simulink model "model_base_2fm"  (R2016b)
settings: Solver=FixedStepDiscrete  StartTime=0.0  StopTime=inf  FixedStep=sampleTime  RelTol=1e-3
PostLoadFcn:
  | % load model parameters
  | base_1fm_parameters;
  | 
  | % set requested state
  | set_param('model_base_2fm/Requested state','Value',num2str(0));
InitFcn:
  | % load model parameters
  | base_1fm_parameters;
  | 
  | % set requested state
  | set_param('model_base_2fm/Requested state','Value',num2str(0));
StartFcn:
  | % load model parameters
  | base_1fm_parameters;
  | 
  | % set requested state
  | set_param('model_base_2fm/Requested state','Value',num2str(0));
undefined symbols (not defined in the file or in its folder): FM1, Lb, Lf, Lu, sampleTime
undefined symbols (not defined in the file): FM2
libraries: simulink x21, LibraryFM x16, VariousBlocksLibrary x4, FMLibrary_v2 x1
(part 1 of 3)
settings Model: SimulationMode=external  Creator=niekbeckers  LastModifiedBy=Labuser
settings DataIOCC: LimitDataPoints=on  SaveFormat=Array
settings OptimizationCC: BlockReduction=off  BooleanDataType=off  LocalBlockOutputs=off  LifeSpan=inf
settings DebuggingCC: SaveWithParameterizedLinksMsg=none  UnderspecifiedInitializationDetection=Classic  MergeDetectMultiDrivingBlocksExec=none  SignalResolutionControl=TryResolveAllWithWarning  SFUnexpectedBacktrackingDiag=warning  SFNoUnconditionalDefaultTransitionDiag=warning  SFExecutionAtInitializationDiag=none
settings HardwareCC: ProdBitPerPointer=32  ProdBitPerSizeT=32  ProdBitPerPtrDiffT=32  ProdLargestAtomicFloat=None  ProdIntDivRoundTo=Undefined  ProdEndianess=Unspecified  ProdWordSize=32  ProdHWDeviceType=32-bit Generic  TargetBitPerPointer=64  TargetBitPerSizeT=64  TargetBitPerPtrDiffT=64  TargetLongLongMode=on  TargetIntDivRoundTo=Zero  TargetEndianess=LittleEndian  TargetWordSize=64  TargetHWDeviceType=MATLAB Host  ProdEqTarget=off
settings ModelReferenceCC: PropagateSignalLabelsOutOfModel=off
settings RTWCC: SystemTargetFile=TwinCAT.tlc  GenCodeOnly=on  MakeCommand=make_tct  TemplateMakefile=tct_msbuild.tmf  Description=TwinCAT Target  GenerateReport=on  TargetLang=C++
settings STFCustomTargetCC: CompOptLevelCompliant=on  GeneratePreprocessorConditionals=Disable all  MATLABClassNameForMDSCustomization=Simulink.SoftwareTarget.TargetSpecificTriggerConfigurationBase  SystemTargetFile=TwinCAT.tlc
settings ConfigComp: CovMetricSettings=dw  CovHtmlReporting=on  CovSaveCumulativeToWorkspaceVar=on  CovSaveSingleToWorkspaceVar=on  CovExternalEMLEnable=off  CovSFcnEnable=off

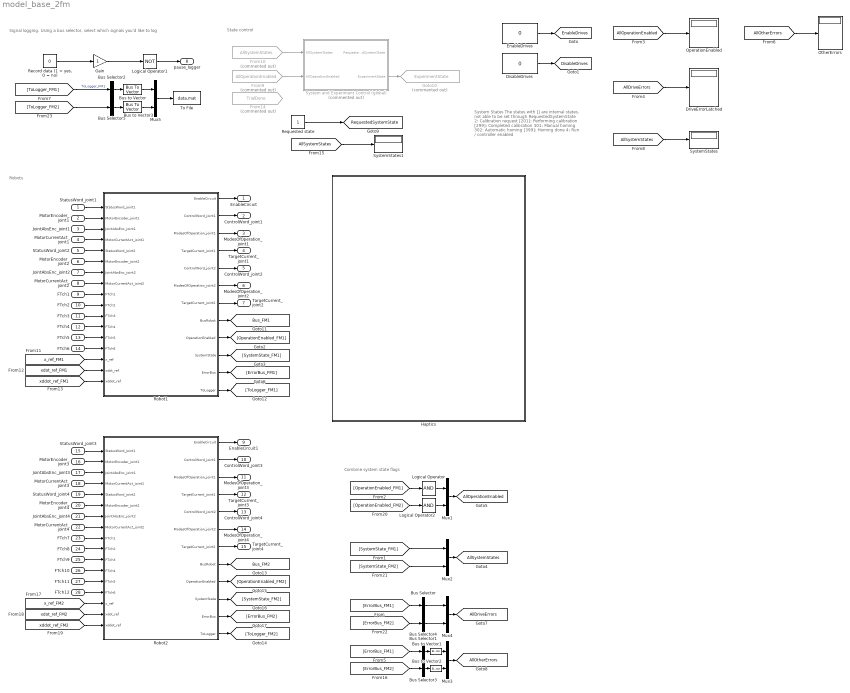
== system model_base_2fm ==
  note: Signal logging.
      | Using a bus selector, select which signals you'd like to log
  note: System States
      | The states with [] are internal states, not able to be set through RequestedSystemState
      | 2: Calibration request
      | [201]: Performing calibration
      | [299]: Completed calibration
      | 301: Manual homing
      | 302: Automatic homing
      | [399]: Homing done
      | 4: Run / controller enabled
  note: State control
  note: Combine system state flags
  note: Robots
  StatusWord_joint1 : Inport  OutDataTypeStr=uint16  PortDimensions=1
  MotorEncoder_joint1 : Inport  Port=2  OutDataTypeStr=int32  PortDimensions=1
  JointAbsEnc_joint1 : Inport  Port=3  OutDataTypeStr=int32  PortDimensions=1
  MotorCurrentAct_joint1 : Inport  Port=4  OutDataTypeStr=int16  PortDimensions=1
  StatusWord_joint2 : Inport  Port=5  OutDataTypeStr=uint16  PortDimensions=1
  MotorEncoder_joint2 : Inport  Port=6  OutDataTypeStr=int32  PortDimensions=1
  JointAbsEnc_joint2 : Inport  Port=7  OutDataTypeStr=int32  PortDimensions=1
  MotorCurrentAct_joint2 : Inport  Port=8  OutDataTypeStr=int16  PortDimensions=1
  FTch1 : Inport  Port=9  OutDataTypeStr=single  PortDimensions=1
  FTch2 : Inport  Port=10  OutDataTypeStr=single  PortDimensions=1
  FTch3 : Inport  Port=11  OutDataTypeStr=single  PortDimensions=1
  FTch4 : Inport  Port=12  OutDataTypeStr=single  PortDimensions=1
  FTch5 : Inport  Port=13  OutDataTypeStr=single  PortDimensions=1
  FTch6 : Inport  Port=14  OutDataTypeStr=single  PortDimensions=1
  StatusWord_joint3 : Inport  Port=15  OutDataTypeStr=uint16  PortDimensions=1
  MotorEncoder_joint3 : Inport  Port=16  OutDataTypeStr=int32  PortDimensions=1
  JointAbsEnc_joint3 : Inport  Port=17  OutDataTypeStr=int32  PortDimensions=1
  MotorCurrentAct_joint3 : Inport  Port=18  OutDataTypeStr=int16  PortDimensions=1
  StatusWord_joint4 : Inport  Port=19  OutDataTypeStr=uint16  PortDimensions=1
  MotorEncoder_joint4 : Inport  Port=20  OutDataTypeStr=int32  PortDimensions=1
  JointAbsEnc_joint4 : Inport  Port=21  OutDataTypeStr=int32  PortDimensions=1
  MotorCurrentAct_joint4 : Inport  Port=22  OutDataTypeStr=int16  PortDimensions=1
  FTch7 : Inport  Port=23  OutDataTypeStr=single  PortDimensions=1
  FTch8 : Inport  Port=24  OutDataTypeStr=single  PortDimensions=1
  FTch9 : Inport  Port=25  OutDataTypeStr=single  PortDimensions=1
  FTch10 : Inport  Port=26  OutDataTypeStr=single  PortDimensions=1
  FTch11 : Inport  Port=27  OutDataTypeStr=single  PortDimensions=1
  FTch12 : Inport  Port=28  OutDataTypeStr=single  PortDimensions=1
  Bus Selector : BusSelector  OutputSignals=DriveErrorLatched  OutputAsBus=on
  Bus Selector1 : BusSelector  OutputSignals=WorkspaceErrorLatched,ForceSensorLatched  OutputAsBus=on
  Bus Selector2 : BusSelector  OutputSignals=SystemState,qJointSpace.q,qJointSpace.qdot,xOpSpace.x,xOpSpace.xdot,Controller_ToLogger.x_ref,Controller_ToLogger.xdot_ref,Controller_ToLogger.xddot_ref,BusFTSensor.ForcesOpSpace,ToEtherCAT_ToLogger_Actuator1.DriveError,ToEtherCAT_ToLogger_Actuator2.DriveError,BusActuators.BusActuator1.JointVelocity_LPF_rads,BusActuators.BusActuator2.JointVelocity_LPF_rads,ToEtherCAT_ToLogger_Actuator1.DesiredTorque_Nm,ToEtherCAT_ToLogger_Actuator2.DesiredTorque_Nm,BusActuators.BusActuator1.JointPosition_AbsEnc_rad,BusActuators.BusActuator2.JointPosition_AbsEnc_rad,BusActuators.BusActuator1.JointVelocity_AbsEnc,BusActuators.BusActuator2.JointVelocity_AbsEnc  OutputAsBus=on
  Bus Selector3 : BusSelector  OutputSignals=WorkspaceErrorLatched,ForceSensorLatched  OutputAsBus=on
  Bus Selector4 : BusSelector  OutputSignals=DriveErrorLatched  OutputAsBus=on
  Bus Selector5 : BusSelector  OutputSignals=SystemState,qJointSpace.q,qJointSpace.qdot,xOpSpace.x,xOpSpace.xdot,Controller_ToLogger.x_ref,Controller_ToLogger.xdot_ref,Controller_ToLogger.xddot_ref,BusFTSensor.ForcesOpSpace,ToEtherCAT_ToLogger_Actuator1.DriveError,ToEtherCAT_ToLogger_Actuator2.DriveError,BusActuators.BusActuator1.JointVelocity_LPF_rads,BusActuators.BusActuator2.JointVelocity_LPF_rads,ToEtherCAT_ToLogger_Actuator1.DesiredTorque_Nm,ToEtherCAT_ToLogger_Actuator2.DesiredTorque_Nm,BusActuators.BusActuator1.JointPosition_AbsEnc_rad,BusActuators.BusActuator2.JointPosition_AbsEnc_rad,BusActuators.BusActuator1.JointVelocity_AbsEnc,BusActuators.BusActuator2.JointVelocity_AbsEnc  OutputAsBus=on
  Bus to Vector{,1..3} (4 alike) : BusToVector
  DisableDrives : Constant  Value=0
      settings: OpenFcn=set_param(gcb,'Value','1');tname = ['toggletimer_' gcb];delete(timerfind('name',tname));t = timer('timerfcn', ['set_param(''',gcb,''',''Value'',''0'')'],'executionmode','singleshot','startdelay',1,'name',tname);start(t);
      mask Display: fprintf('PushToTrigger\n%s',get_param(gcb,'value'))
  DriveErrorLatched : Display
  EnableDrives : Constant  Value=0
      settings: OpenFcn=set_param(gcb,'Value','1');tname = ['toggletimer_' gcb];delete(timerfind('name',tname));t = timer('timerfcn', ['set_param(''',gcb,''',''Value'',''0'')'],'executionmode','singleshot','startdelay',1,'name',tname);start(t);
      mask Display: fprintf('PushToTrigger\n%s',get_param(gcb,'value'))
  From10 : From  Commented=on  GotoTag=AllSystemStates
  From14 : From  Commented=on  GotoTag=TrialDone
  From9 : From  Commented=on  GotoTag=AllOperationEnabled
  Gain : Gain
  Goto10 : Goto  Commented=on  GotoTag=ExperimentState  TagVisibility=global
  Haptics : Subsystem
  Logical Operator : Logic  Inputs=1  AllPortsSameDT=off  OutDataTypeStr=boolean
  Logical Operator1 : Logic  Operator=NOT  Inputs=1  AllPortsSameDT=off  OutDataTypeStr=boolean
  Logical Operator2 : Logic  Inputs=1  AllPortsSameDT=off  OutDataTypeStr=boolean
  Mux{1..5} (5 alike) : Mux  Inputs=2
  OperationEnabled : Display
  OtherErrors : Display
  "Record data (1 = yes, 0 = no)" : Constant  Value=0
  Requested state : Constant
  Robot1 : Subsystem  mask{RobotStruct=FM1}
      mask prompts: RobotStruct "Robot struct (data)"
  Robot2 : Subsystem  mask{RobotStruct=FM2}
      mask prompts: RobotStruct "Robot struct (data)"
  System and Experiment Control (global) : Subsystem  Commented=on
  SystemStates : Display
  SystemStates1 : Display
  To File : ToFile  Filename=data.mat  MatrixName=data
  EnableCircuit : Outport  OutDataTypeStr=boolean  PortDimensions=1
  ControlWord_joint1 : Outport  Port=2  OutDataTypeStr=uint16  PortDimensions=1
  ModesOfOperation_joint1 : Outport  Port=3  OutDataTypeStr=int8  PortDimensions=1
  TargetCurrent_joint1 : Outport  Port=4  OutDataTypeStr=int16  PortDimensions=1
  ControlWord_joint2 : Outport  Port=5  OutDataTypeStr=uint16  PortDimensions=1
  ModesOfOperation_joint2 : Outport  Port=6  OutDataTypeStr=int8  PortDimensions=1
  TargetCurrent_joint2 : Outport  Port=7  OutDataTypeStr=int16  PortDimensions=1
  pause_logger : Outport  Port=8  OutDataTypeStr=boolean  PortDimensions=1
  EnableCircuit1 : Outport  Port=9  OutDataTypeStr=boolean  PortDimensions=1
  ControlWord_joint3 : Outport  Port=10  OutDataTypeStr=uint16  PortDimensions=1
  ModesOfOperation_joint3 : Outport  Port=11  OutDataTypeStr=int8  PortDimensions=1
  TargetCurrent_joint3 : Outport  Port=12  OutDataTypeStr=int16  PortDimensions=1
  ControlWord_joint4 : Outport  Port=13  OutDataTypeStr=uint16  PortDimensions=1
  ModesOfOperation_joint4 : Outport  Port=14  OutDataTypeStr=int8  PortDimensions=1
  TargetCurrent_joint4 : Outport  Port=15  OutDataTypeStr=int16  PortDimensions=1
  tag scope: AllDriveErrors=global, AllOperationEnabled=global, AllOtherErrors=global, AllSystemStates=global, Bus_FM1=global, Bus_FM2=global, DisableDrives=global, EnableDrives=global, RequestedSystemState=global
  wires:
  DisableDrives/1 -> [DisableDrives]
  EnableDrives/1 -> [EnableDrives]
  Robot1/9(OperationEnabled) -> [OperationEnabled_FM1]
  [AllOperationEnabled] -> OperationEnabled/1
  Robot1/10(SystemState) -> [SystemState_FM1]
  [SystemState_FM1] -> Mux2/1
  Mux2/1 -> [AllSystemStates]
  Mux1/1 -> [AllOperationEnabled]
  [OperationEnabled_FM1] -> Logical Operator/1
  Robot1/11(ErrorBus) -> [ErrorBus_FM1]
  [ErrorBus_FM1] -> Bus Selector/1
  [AllDriveErrors] -> DriveErrorLatched/1
  [ErrorBus_FM1] -> Bus Selector1/1
  [AllOtherErrors] -> OtherErrors/1
  [AllSystemStates] -> SystemStates/1
  System and Experiment Control (global)/2(ExperimentState) -> Goto10/1
  From10/1 -> System and Experiment Control (global)/1(AllSystemStates)
  From9/1 -> System and Experiment Control (global)/2(AllOperationEnabled)
  [x_ref_FM1] -> Robot1/15(x_ref)
  [xdot_ref_FM1] -> Robot1/16(xdot_ref)
  [xddot_ref_FM1] -> Robot1/17(xddot_ref)
  Requested state/1 -> [RequestedSystemState]
  Robot1/8(BusRobot) -> [Bus_FM1]
  StatusWord_joint1/1 -> Robot1/1(StatusWord_joint1)
  MotorEncoder_joint1/1 -> Robot1/2(MotorEncoder_joint1)
  JointAbsEnc_joint1/1 -> Robot1/3(JointAbsEnc_joint1)
  MotorCurrentAct_joint1/1 -> Robot1/4(MotorCurrentAct_joint1)
  StatusWord_joint2/1 -> Robot1/5(StatusWord_joint2)
  MotorEncoder_joint2/1 -> Robot1/6(MotorEncoder_joint2)
  JointAbsEnc_joint2/1 -> Robot1/7(JointAbsEnc_joint2)
  MotorCurrentAct_joint2/1 -> Robot1/8(MotorCurrentAct_joint2)
  FTch1/1 -> Robot1/9(FTch1)
  FTch2/1 -> Robot1/10(FTch2)
  FTch3/1 -> Robot1/11(FTch3)
  FTch4/1 -> Robot1/12(FTch4)
  FTch5/1 -> Robot1/13(FTch5)
  FTch6/1 -> Robot1/14(FTch6)
  Robot1/1(EnableCircuit) -> EnableCircuit/1
  Robot1/2(ControlWord_joint1) -> ControlWord_joint1/1
  Robot1/3(ModesOfOperation_joint1) -> ModesOfOperation_joint1/1
  Robot1/4(TargetCurrent_joint1) -> TargetCurrent_joint1/1
  Robot1/7(TargetCurrent_joint2) -> TargetCurrent_joint2/1
  Robot1/6(ModesOfOperation_joint2) -> ModesOfOperation_joint2/1
  Robot1/5(ControlWord_joint2) -> ControlWord_joint2/1
  Robot1/12(ToLogger) -> [ToLogger_FM1]
  [ToLogger_FM1] -> Bus Selector2/1  "ToLogger_FM1"
  Logical Operator/1 -> Mux1/1
  [AllSystemStates] -> SystemStates1/1
  Logical Operator1/1 -> pause_logger/1
  Bus Selector2/1 -> Bus to Vector/1
  "Record data (1 = yes, 0 = no)"/1 -> Gain/1
  Robot2/9(OperationEnabled) -> [OperationEnabled_FM2]
  Robot2/10(SystemState) -> [SystemState_FM2]
  Robot2/11(ErrorBus) -> [ErrorBus_FM2]
  [x_ref_FM2] -> Robot2/15(x_ref)
  [xdot_ref_FM2] -> Robot2/16(xdot_ref)
  [xddot_ref_FM2] -> Robot2/17(xddot_ref)
  Robot2/8(BusRobot) -> [Bus_FM2]
  StatusWord_joint3/1 -> Robot2/1(StatusWord_joint1)
  MotorEncoder_joint3/1 -> Robot2/2(MotorEncoder_joint1)
  JointAbsEnc_joint3/1 -> Robot2/3(JointAbsEnc_joint1)
  MotorCurrentAct_joint3/1 -> Robot2/4(MotorCurrentAct_joint1)
  StatusWord_joint4/1 -> Robot2/5(StatusWord_joint2)
  MotorEncoder_joint4/1 -> Robot2/6(MotorEncoder_joint2)
  JointAbsEnc_joint4/1 -> Robot2/7(JointAbsEnc_joint2)
  MotorCurrentAct_joint4/1 -> Robot2/8(MotorCurrentAct_joint2)
  FTch7/1 -> Robot2/9(FTch1)
  FTch8/1 -> Robot2/10(FTch2)
  FTch9/1 -> Robot2/11(FTch3)
  FTch10/1 -> Robot2/12(FTch4)
  FTch11/1 -> Robot2/13(FTch5)
  FTch12/1 -> Robot2/14(FTch6)
  Robot2/1(EnableCircuit) -> EnableCircuit1/1
  Robot2/2(ControlWord_joint1) -> ControlWord_joint3/1
  Robot2/3(ModesOfOperation_joint1) -> ModesOfOperation_joint3/1
  Robot2/4(TargetCurrent_joint1) -> TargetCurrent_joint3/1
  Robot2/7(TargetCurrent_joint2) -> TargetCurrent_joint4/1
  Robot2/6(ModesOfOperation_joint2) -> ModesOfOperation_joint4/1
  Robot2/5(ControlWord_joint2) -> ControlWord_joint4/1
  Robot2/12(ToLogger) -> [ToLogger_FM2]
  [OperationEnabled_FM2] -> Logical Operator2/1
  Logical Operator2/1 -> Mux1/2
  [SystemState_FM2] -> Mux2/2
  [ErrorBus_FM2] -> Bus Selector3/1
  Bus Selector1/1 -> Bus to Vector1/1
  Mux3/1 -> [AllOtherErrors]
  Bus to Vector1/1 -> Mux3/1
  Bus Selector3/1 -> Bus to Vector2/1
  Bus to Vector2/1 -> Mux3/2
  Mux4/1 -> [AllDriveErrors]
  Bus Selector/1 -> Mux4/1
  [ErrorBus_FM2] -> Bus Selector4/1
  Bus Selector4/1 -> Mux4/2
  [ToLogger_FM2] -> Bus Selector5/1
  Bus Selector5/1 -> Bus to Vector3/1
  Bus to Vector3/1 -> Mux5/2
  Bus to Vector/1 -> Mux5/1
  Mux5/1 -> To File/1
  Gain/1 -> Logical Operator1/1

== system model_base_2fm/Haptics ==
  note: Only run trajectory if all systems are in state 4 (run)
  Add : Sum  Commented=on
  Bus Selector : BusSelector  OutputSignals=xOpSpace.x,xOpSpace.xdot
  Bus Selector1 : BusSelector  OutputSignals=xOpSpace.x,xOpSpace.xdot
  "Check state " : simulink/Logic and Bit Operations/Compare To Constant  Commented=on  relop===  const=4  OutDataTypeStr=boolean
  Constant : Constant  Commented=on  Value=FM1.HomeLocationOpSpace
  Constant1 : Constant  Value=[0;0]
  From9 : From  Commented=on  GotoTag=ExperimentState
  Goto1 : Goto  Commented=on  GotoTag=TrialDone  TagVisibility=global
  Hypotrochoid trajectory for AFFC : Subsystem  Commented=on
  Logical Operator : Logic  Commented=on  Inputs=1  AllPortsSameDT=off  OutDataTypeStr=boolean
  Terminator1 : Terminator  Commented=on
  Terminator2 : Terminator  Commented=on
  tag scope: x_ref_FM1=global, x_ref_FM2=global, xddot_ref_FM1=global, xddot_ref_FM2=global, xdot_ref_FM1=global, xdot_ref_FM2=global
  wires:
  From9/1 -> Terminator1/1
  [Bus_FM1] -> Bus Selector/1
  Constant/1 -> Add/1
  Hypotrochoid trajectory for AFFC/1(dx_ref) -> Add/2
  Add/1 -> ?
  Hypotrochoid trajectory for AFFC/2(dxdot_ref) -> ?
  Hypotrochoid trajectory for AFFC/3(dxddot_ref) -> ?
  ? -> "Check state "/1
  "Check state "/1 -> Logical Operator/1
  Logical Operator/1 -> Hypotrochoid trajectory for AFFC/Enable
  [Bus_FM2] -> Bus Selector1/1
  Constant1/1 -> [xddot_ref_FM2], [xddot_ref_FM1]
  Bus Selector/1 -> [x_ref_FM2]  "<x>"
  Bus Selector/2 -> [xdot_ref_FM2]  "<xdot>"
  Bus Selector1/2 -> [xdot_ref_FM1]  "<xdot>"
  Bus Selector1/1 -> [x_ref_FM1]  "<x>"
  [AllSystemStates] -> Terminator2/1

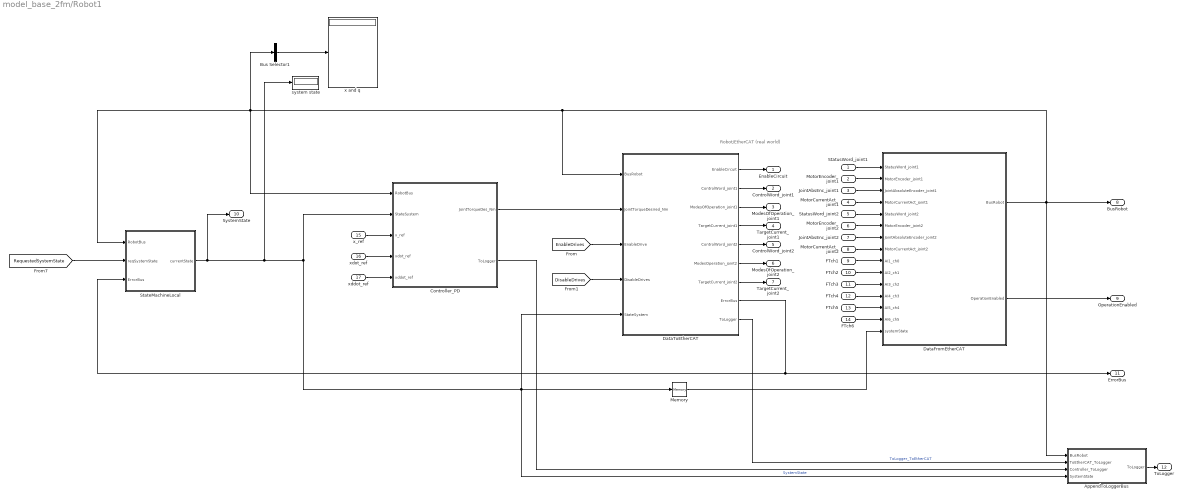
== system model_base_2fm/Robot1 ==
  note: Robot/EtherCAT (real world)
  StatusWord_joint1 : Inport
  MotorEncoder_joint1 : Inport  Port=2
  JointAbsEnc_joint1 : Inport  Port=3
  MotorCurrentAct_joint1 : Inport  Port=4
  StatusWord_joint2 : Inport  Port=5
  MotorEncoder_joint2 : Inport  Port=6
  JointAbsEnc_joint2 : Inport  Port=7
  MotorCurrentAct_joint2 : Inport  Port=8
  FTch1 : Inport  Port=9
  FTch2 : Inport  Port=10
  FTch3 : Inport  Port=11
  FTch4 : Inport  Port=12
  FTch5 : Inport  Port=13
  FTch6 : Inport  Port=14
  x_ref : Inport  Port=15
  xdot_ref : Inport  Port=16
  xddot_ref : Inport  Port=17
  AppendToLoggerBus : Subsystem
  Bus Selector1 : BusSelector  OutputSignals=qJointSpace.q,qJointSpace.qdot,xOpSpace.x,BusActuators.BusActuator1.JointPosition_AbsEnc_rad,BusActuators.BusActuator2.JointPosition_AbsEnc_rad  OutputAsBus=on
  Controller_PD : Subsystem
  DataFromEtherCAT : Subsystem
  DataToEtherCAT : Subsystem
  Memory : Memory
  StateMachineLocal : Subsystem
  system state : Display
  x and q : Display
  EnableCircuit : Outport
  ControlWord_joint1 : Outport  Port=2
  ModesOfOperation_joint1 : Outport  Port=3
  TargetCurrent_joint1 : Outport  Port=4
  ControlWord_joint2 : Outport  Port=5
  ModesOfOperation_joint2 : Outport  Port=6
  TargetCurrent_joint2 : Outport  Port=7
  BusRobot : Outport  Port=8
  OperationEnabled : Outport  Port=9
  SystemState : Outport  Port=10
  ErrorBus : Outport  Port=11
  ToLogger : Outport  Port=12
  wires:
  xddot_ref/1 -> Controller_PD/5(xddot_ref)
  xdot_ref/1 -> Controller_PD/4(xdot_ref)
  x_ref/1 -> Controller_PD/3(x_ref)
  DataToEtherCAT/7(TargetCurrent_joint2) -> TargetCurrent_joint2/1
  FTch2/1 -> DataFromEtherCAT/10(AI2_ch1)
  MotorCurrentAct_joint1/1 -> DataFromEtherCAT/4(MotorCurrentAct_joint1)
  MotorEncoder_joint2/1 -> DataFromEtherCAT/6(MotorEncoder_joint2)
  JointAbsEnc_joint1/1 -> DataFromEtherCAT/3(JointAbsoluteEncoder_joint1)
  DataToEtherCAT/3(ModesOfOperation_joint1) -> ModesOfOperation_joint1/1
  DataToEtherCAT/1(EnableCircuit) -> EnableCircuit/1
  FTch1/1 -> DataFromEtherCAT/9(AI1_ch0)
  StateMachineLocal/1(currentState) -> system state/1, DataToEtherCAT/5(StateSystem), Memory/1, AppendToLoggerBus/4(SystemState), Controller_PD/2(StateSystem), SystemState/1  "SystemState"
  DataToEtherCAT/2(ControlWord_joint1) -> ControlWord_joint1/1
  DataToEtherCAT/8(ErrorBus) -> StateMachineLocal/3(ErrorBus), ErrorBus/1
  DataFromEtherCAT/1(BusRobot) -> AppendToLoggerBus/1(BusRobot), Controller_PD/1(RobotBus), Bus Selector1/1, StateMachineLocal/1(RobotBus), DataToEtherCAT/1(BusRobot), BusRobot/1
  [RequestedSystemState] -> StateMachineLocal/2(reqSystemState)
  Controller_PD/1(JointTorqueDes_Nm) -> DataToEtherCAT/2(JointTorqueDesired_Nm)
  [DisableDrives] -> DataToEtherCAT/4(DisableDrives)
  [EnableDrives] -> DataToEtherCAT/3(EnableDrive)
  MotorCurrentAct_joint2/1 -> DataFromEtherCAT/8(MotorCurrentAct_joint2)
  DataToEtherCAT/4(TargetCurrent_joint1) -> TargetCurrent_joint1/1
  FTch5/1 -> DataFromEtherCAT/13(AI5_ch4)
  JointAbsEnc_joint2/1 -> DataFromEtherCAT/7("JointAbsoluteEncoder_joint2 ")
  MotorEncoder_joint1/1 -> DataFromEtherCAT/2(MotorEncoder_joint1)
  DataToEtherCAT/5(ControlWord_joint2) -> ControlWord_joint2/1
  DataToEtherCAT/6(ModesOperation_joint2) -> ModesOfOperation_joint2/1
  StatusWord_joint1/1 -> DataFromEtherCAT/1(StatusWord_joint1)
  StatusWord_joint2/1 -> DataFromEtherCAT/5(StatusWord_joint2)
  FTch6/1 -> DataFromEtherCAT/14(AI6_ch5)
  FTch4/1 -> DataFromEtherCAT/12(AI4_ch3)
  FTch3/1 -> DataFromEtherCAT/11(AI3_ch2)
  DataFromEtherCAT/2(OperationEnabled) -> OperationEnabled/1
  Bus Selector1/1 -> x and q/1
  Controller_PD/2(ToLogger) -> AppendToLoggerBus/3(Controller_ToLogger)
  DataToEtherCAT/9(ToLogger) -> AppendToLoggerBus/2(ToEtherCAT_ToLogger)  "ToLogger_ToEtherCAT"
  AppendToLoggerBus/1(ToLogger) -> ToLogger/1
  Memory/1 -> DataFromEtherCAT/15(systemState)

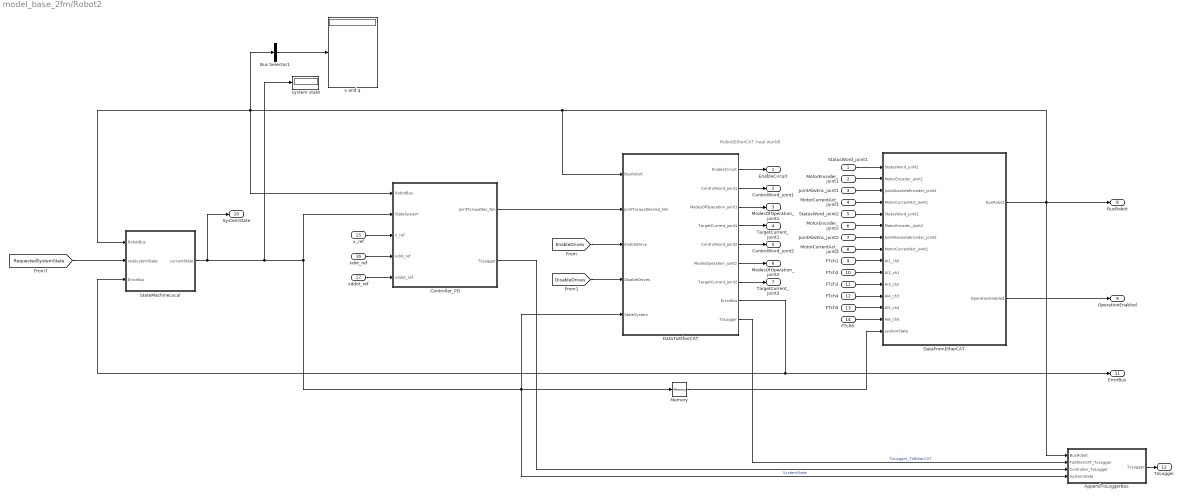
== system model_base_2fm/Robot2 ==
  note: Robot/EtherCAT (real world)
  StatusWord_joint1 : Inport
  MotorEncoder_joint1 : Inport  Port=2
  JointAbsEnc_joint1 : Inport  Port=3
  MotorCurrentAct_joint1 : Inport  Port=4
  StatusWord_joint2 : Inport  Port=5
  MotorEncoder_joint2 : Inport  Port=6
  JointAbsEnc_joint2 : Inport  Port=7
  MotorCurrentAct_joint2 : Inport  Port=8
  FTch1 : Inport  Port=9
  FTch2 : Inport  Port=10
  FTch3 : Inport  Port=11
  FTch4 : Inport  Port=12
  FTch5 : Inport  Port=13
  FTch6 : Inport  Port=14
  x_ref : Inport  Port=15
  xdot_ref : Inport  Port=16
  xddot_ref : Inport  Port=17
  AppendToLoggerBus : Subsystem
  Bus Selector1 : BusSelector  OutputSignals=qJointSpace.q,qJointSpace.qdot,xOpSpace.x,BusActuators.BusActuator1.JointPosition_AbsEnc_rad,BusActuators.BusActuator2.JointPosition_AbsEnc_rad  OutputAsBus=on
  Controller_PD : Subsystem
  DataFromEtherCAT : Subsystem
  DataToEtherCAT : Subsystem
  Memory : Memory
  StateMachineLocal : Subsystem
  system state : Display
  x and q : Display
  EnableCircuit : Outport
  ControlWord_joint1 : Outport  Port=2
  ModesOfOperation_joint1 : Outport  Port=3
  TargetCurrent_joint1 : Outport  Port=4
  ControlWord_joint2 : Outport  Port=5
  ModesOfOperation_joint2 : Outport  Port=6
  TargetCurrent_joint2 : Outport  Port=7
  BusRobot : Outport  Port=8
  OperationEnabled : Outport  Port=9
  SystemState : Outport  Port=10
  ErrorBus : Outport  Port=11
  ToLogger : Outport  Port=12
  wires:
  xddot_ref/1 -> Controller_PD/5(xddot_ref)
  xdot_ref/1 -> Controller_PD/4(xdot_ref)
  x_ref/1 -> Controller_PD/3(x_ref)
  DataToEtherCAT/7(TargetCurrent_joint2) -> TargetCurrent_joint2/1
  FTch2/1 -> DataFromEtherCAT/10(AI2_ch1)
  MotorCurrentAct_joint1/1 -> DataFromEtherCAT/4(MotorCurrentAct_joint1)
  MotorEncoder_joint2/1 -> DataFromEtherCAT/6(MotorEncoder_joint2)
  JointAbsEnc_joint1/1 -> DataFromEtherCAT/3(JointAbsoluteEncoder_joint1)
  DataToEtherCAT/3(ModesOfOperation_joint1) -> ModesOfOperation_joint1/1
  DataToEtherCAT/1(EnableCircuit) -> EnableCircuit/1
  FTch1/1 -> DataFromEtherCAT/9(AI1_ch0)
  StateMachineLocal/1(currentState) -> system state/1, DataToEtherCAT/5(StateSystem), Memory/1, AppendToLoggerBus/4(SystemState), Controller_PD/2(StateSystem), SystemState/1  "SystemState"
  DataToEtherCAT/2(ControlWord_joint1) -> ControlWord_joint1/1
  DataToEtherCAT/8(ErrorBus) -> StateMachineLocal/3(ErrorBus), ErrorBus/1
  DataFromEtherCAT/1(BusRobot) -> AppendToLoggerBus/1(BusRobot), Controller_PD/1(RobotBus), Bus Selector1/1, StateMachineLocal/1(RobotBus), DataToEtherCAT/1(BusRobot), BusRobot/1
  [RequestedSystemState] -> StateMachineLocal/2(reqSystemState)
  Controller_PD/1(JointTorqueDes_Nm) -> DataToEtherCAT/2(JointTorqueDesired_Nm)
  [DisableDrives] -> DataToEtherCAT/4(DisableDrives)
  [EnableDrives] -> DataToEtherCAT/3(EnableDrive)
  MotorCurrentAct_joint2/1 -> DataFromEtherCAT/8(MotorCurrentAct_joint2)
  DataToEtherCAT/4(TargetCurrent_joint1) -> TargetCurrent_joint1/1
  FTch5/1 -> DataFromEtherCAT/13(AI5_ch4)
  JointAbsEnc_joint2/1 -> DataFromEtherCAT/7("JointAbsoluteEncoder_joint2 ")
  MotorEncoder_joint1/1 -> DataFromEtherCAT/2(MotorEncoder_joint1)
  DataToEtherCAT/5(ControlWord_joint2) -> ControlWord_joint2/1
  DataToEtherCAT/6(ModesOperation_joint2) -> ModesOfOperation_joint2/1
  StatusWord_joint1/1 -> DataFromEtherCAT/1(StatusWord_joint1)
  StatusWord_joint2/1 -> DataFromEtherCAT/5(StatusWord_joint2)
  FTch6/1 -> DataFromEtherCAT/14(AI6_ch5)
  FTch4/1 -> DataFromEtherCAT/12(AI4_ch3)
  FTch3/1 -> DataFromEtherCAT/11(AI3_ch2)
  DataFromEtherCAT/2(OperationEnabled) -> OperationEnabled/1
  Bus Selector1/1 -> x and q/1
  Controller_PD/2(ToLogger) -> AppendToLoggerBus/3(Controller_ToLogger)
  DataToEtherCAT/9(ToLogger) -> AppendToLoggerBus/2(ToEtherCAT_ToLogger)  "ToLogger_ToEtherCAT"
  AppendToLoggerBus/1(ToLogger) -> ToLogger/1
  Memory/1 -> DataFromEtherCAT/15(systemState)

== system model_base_2fm/System and Experiment Control (global) ==
  note: Hier ergens experiment protocol inlezen
  AllSystemStates : Inport
  AllOperationEnabled : Inport  Port=2
  GlobalStateMachine : FMLibrary_v2/StateMachineLocal/SystemLocalStateMachine
  RequestedSystemState : Outport
  ExperimentState : Outport  Port=2
  wires:
  GlobalStateMachine/1 -> RequestedSystemState/1

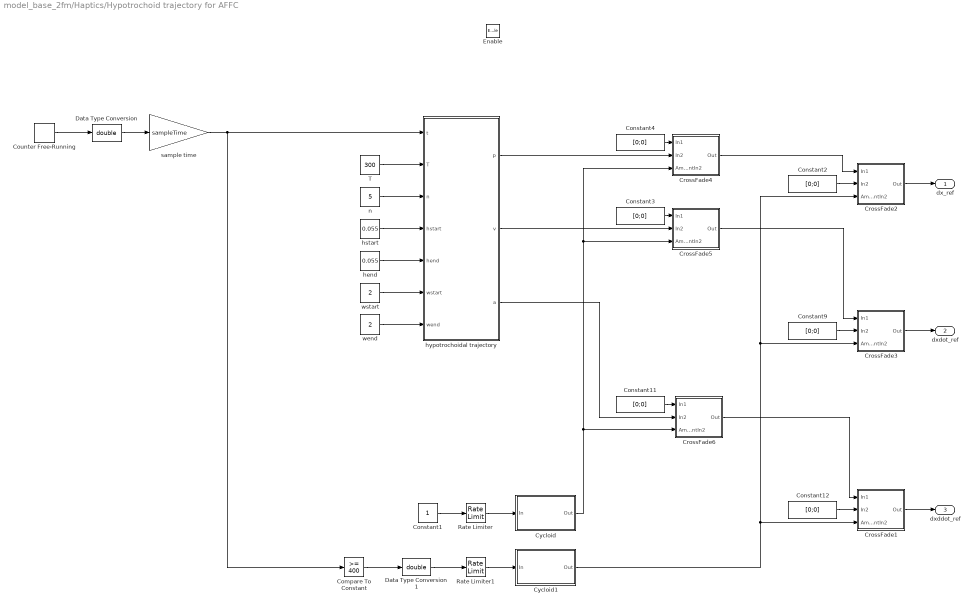
== system model_base_2fm/Haptics/Hypotrochoid trajectory for AFFC ==
  Enable : EnablePort  StatesWhenEnabling=reset
  Compare To Constant : simulink/Logic and Bit Operations/Compare To Constant  relop=>=  const=400  OutDataTypeStr=boolean
  Constant1 : Constant
  Constant{2..4,9,11..12} (6 alike) : Constant  Value=[0;0]
  Counter Free-Running : simulink/Sources/Counter Free-Running  NumBits=32  tsamp=-1
  CrossFade1 : Subsystem  AncestorBlock=VariousBlocksLibrary/Various/CrossFade
  CrossFade2 : Subsystem  AncestorBlock=VariousBlocksLibrary/Various/CrossFade
  CrossFade3 : Subsystem  AncestorBlock=VariousBlocksLibrary/Various/CrossFade
  CrossFade4 : Subsystem
  CrossFade5 : Subsystem  AncestorBlock=VariousBlocksLibrary/Various/CrossFade
  CrossFade6 : Subsystem  AncestorBlock=VariousBlocksLibrary/Various/CrossFade
  Cycloid : Subsystem  AncestorBlock=VariousBlocksLibrary/Various/Cycloid
  Cycloid1 : Subsystem  AncestorBlock=VariousBlocksLibrary/Various/Cycloid
  Data Type Conversion : DataTypeConversion  OutDataTypeStr=double
  Data Type Conversion1 : DataTypeConversion  OutDataTypeStr=double
  Rate Limiter : RateLimiter  RisingSlewLimit=0.25  FallingSlewLimit=-0.15  SampleTimeMode=inherited
  Rate Limiter1 : RateLimiter  RisingSlewLimit=0.2  FallingSlewLimit=-0.2  SampleTimeMode=inherited
  T : Constant  Value=300
  hend : Constant  Value=0.055
  hstart : Constant  Value=0.055
  hypotrochoidal trajectory : MATLAB Function  TreatAsAtomicUnit=on
  n : Constant  Value=5
  sample time : Gain  Gain=sampleTime
  wend : Constant  Value=2
  wstart : Constant  Value=2
  dx_ref : Outport  InitialOutput=[0;0]
  dxdot_ref : Outport  Port=2  InitialOutput=[0;0]
  dxddot_ref : Outport  Port=3  InitialOutput=[0;0]
  wires:
  Data Type Conversion1/1 -> Rate Limiter1/1
  hypotrochoidal trajectory/1(p) -> CrossFade4/2(In2)
  CrossFade1/1(Out) -> dxddot_ref/1
  Constant11/1 -> CrossFade6/1(In1)
  Constant12/1 -> CrossFade1/2(In2)
  CrossFade6/1(Out) -> CrossFade1/1(In1)
  Constant9/1 -> CrossFade3/2(In2)
  CrossFade5/1(Out) -> CrossFade3/1(In1)
  CrossFade3/1(Out) -> dxdot_ref/1
  Cycloid1/1(Out) -> CrossFade1/3(AmountIn2), CrossFade2/3(AmountIn2), CrossFade3/3(AmountIn2)
  Rate Limiter1/1 -> Cycloid1/1(In)
  Compare To Constant/1 -> Data Type Conversion1/1
  CrossFade4/1(Out) -> CrossFade2/1(In1)
  CrossFade2/1(Out) -> dx_ref/1
  Rate Limiter/1 -> Cycloid/1(In)
  Constant1/1 -> Rate Limiter/1
  Cycloid/1(Out) -> CrossFade6/3(AmountIn2), CrossFade5/3(AmountIn2), CrossFade4/3(AmountIn2)
  hypotrochoidal trajectory/2(v) -> CrossFade5/2(In2)
  hypotrochoidal trajectory/3(a) -> CrossFade6/2(In2)
  sample time/1 -> Compare To Constant/1, hypotrochoidal trajectory/1(t)
  Constant2/1 -> CrossFade2/2(In2)
  Data Type Conversion/1 -> sample time/1
  wstart/1 -> hypotrochoidal trajectory/6(wstart)
  wend/1 -> hypotrochoidal trajectory/7(wend)
  hstart/1 -> hypotrochoidal trajectory/4(hstart)
  hend/1 -> hypotrochoidal trajectory/5(hend)
  n/1 -> hypotrochoidal trajectory/3(n)
  T/1 -> hypotrochoidal trajectory/2(T)
  Counter Free-Running/1 -> Data Type Conversion/1
  Constant3/1 -> CrossFade5/1(In1)
  Constant4/1 -> CrossFade4/1(In1)

== system model_base_2fm/Robot1/AppendToLoggerBus ==
  BusRobot : Inport
  ToEtherCAT_ToLogger : Inport  Port=2
  Controller_ToLogger : Inport  Port=3
  SystemState : Inport  Port=4
  Bus Creator : BusCreator  Inputs=8
  Bus Selector : BusSelector  OutputSignals=xOpSpace,qJointSpace,BusFTSensor,BusActuators
  Bus Selector1 : BusSelector  OutputSignals=ToEtherCAT_ToLogger_Actuator1,ToEtherCAT_ToLogger_Actuator2
  ToLogger : Outport
  wires:
  Bus Creator/1 -> ToLogger/1  "LoggerBus"
  Bus Selector/4 -> Bus Creator/4  "<BusActuators>"
  Bus Selector/1 -> Bus Creator/1  "<xOpSpace>"
  Bus Selector/3 -> Bus Creator/3  "<BusFTSensor>"
  Bus Selector/2 -> Bus Creator/2  "<qJointSpace>"
  BusRobot/1 -> Bus Selector/1
  ToEtherCAT_ToLogger/1 -> Bus Selector1/1
  Bus Selector1/1 -> Bus Creator/5  "<ToEtherCAT_ToLogger_Actuator1>"
  Bus Selector1/2 -> Bus Creator/6  "<ToEtherCAT_ToLogger_Actuator2>"
  Controller_ToLogger/1 -> Bus Creator/7
  SystemState/1 -> Bus Creator/8  "SystemState"

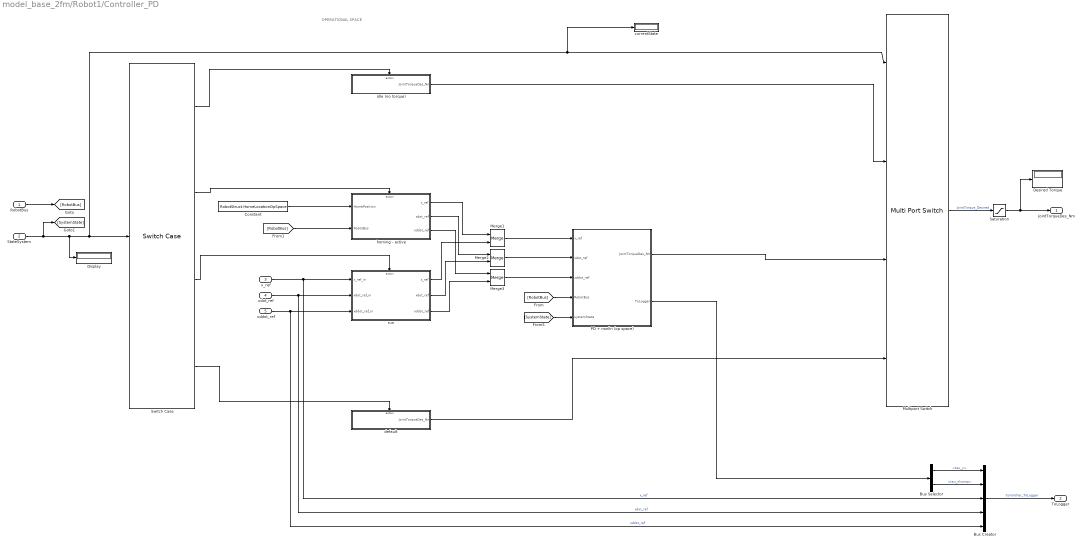
== system model_base_2fm/Robot1/Controller_PD ==
  note: OPERATIONAL SPACE
  RobotBus : Inport
  StateSystem : Inport  Port=2
  x_ref : Inport  Port=3
  xdot_ref : Inport  Port=4
  xddot_ref : Inport  Port=5
  Bus Creator : BusCreator  Inputs=5
  Bus Selector : BusSelector  OutputSignals=tau_y,tau_nlcomp
  Constant : Constant  Value=RobotStruct.HomeLocationOpSpace
  Desired Torque : Display
  Display : Display
  Merge1 : Merge  InitialOutput=[0;0]
  Merge2 : Merge  InitialOutput=[0;0]
  Merge3 : Merge  InitialOutput=[0;0]
  Multiport Switch : MultiPortSwitch  DataPortOrder=Specify indices  Inputs=4  DataPortIndices={[0,1,2,201,299,301],[302,399,4]}  DataPortForDefault=Additional data port
  PD + nonlin (op space) : Subsystem
  Saturation : Saturate  UpperLimit=4  LowerLimit=-4
  Switch Case : SwitchCase  CaseConditions={[0,1,2,201,299,301],[302, 399],[4]}
  currentState : Display
  default : Subsystem  TreatAsAtomicUnit=on
  homing - active : Subsystem
  idle (no torque) : Subsystem  TreatAsAtomicUnit=on
  run : Subsystem
  JointTorqueDes_Nm : Outport
  ToLogger : Outport  Port=2
  wires:
  [SystemState] -> PD + nonlin (op space)/5(systemState)
  xddot_ref/1 -> Bus Creator/5, run/3(xddot_ref_in)  "xddot_ref"
  xdot_ref/1 -> Bus Creator/4, run/2(xdot_ref_in)  "xdot_ref"
  x_ref/1 -> Bus Creator/3, run/1(x_ref_in)  "x_ref"
  [RobotBus] -> homing - active/2(RobotBus)
  [RobotBus] -> PD + nonlin (op space)/4(RobotBus)
  RobotBus/1 -> [RobotBus]
  PD + nonlin (op space)/1(JointTorqueDes_Nm) -> Multiport Switch/3
  Merge3/1 -> PD + nonlin (op space)/3(xddot_ref)
  Merge2/1 -> PD + nonlin (op space)/2(xdot_ref)
  Merge1/1 -> PD + nonlin (op space)/1(x_ref)
  idle (no torque)/1(JointTorqueDes_Nm) -> Multiport Switch/2
  Switch Case/2 -> homing - active/Action
  Switch Case/1 -> idle (no torque)/Action
  default/1(JointTorqueDes_Nm) -> Multiport Switch/4
  Switch Case/4 -> default/Action
  Saturation/1 -> Desired Torque/1, JointTorqueDes_Nm/1
  Switch Case/3 -> run/Action
  homing - active/1(x_ref) -> Merge1/1
  run/1(x_ref) -> Merge1/2
  StateSystem/1 -> Display/1, Multiport Switch/1, currentState/1, Switch Case/1, [SystemState]
  run/2(xdot_ref) -> Merge2/2
  run/3(xddot_ref) -> Merge3/2
  homing - active/2(xdot_ref) -> Merge2/1
  homing - active/3(xddot_ref) -> Merge3/1
  Multiport Switch/1 -> Saturation/1  "JointTorque_Desired"
  PD + nonlin (op space)/2(ToLogger) -> Bus Selector/1
  Constant/1 -> homing - active/1(HomePosition)
  Bus Creator/1 -> ToLogger/1  "Controller_ToLogger"
  Bus Selector/1 -> Bus Creator/1  "<tau_y>"
  Bus Selector/2 -> Bus Creator/2  "<tau_nlcomp>"

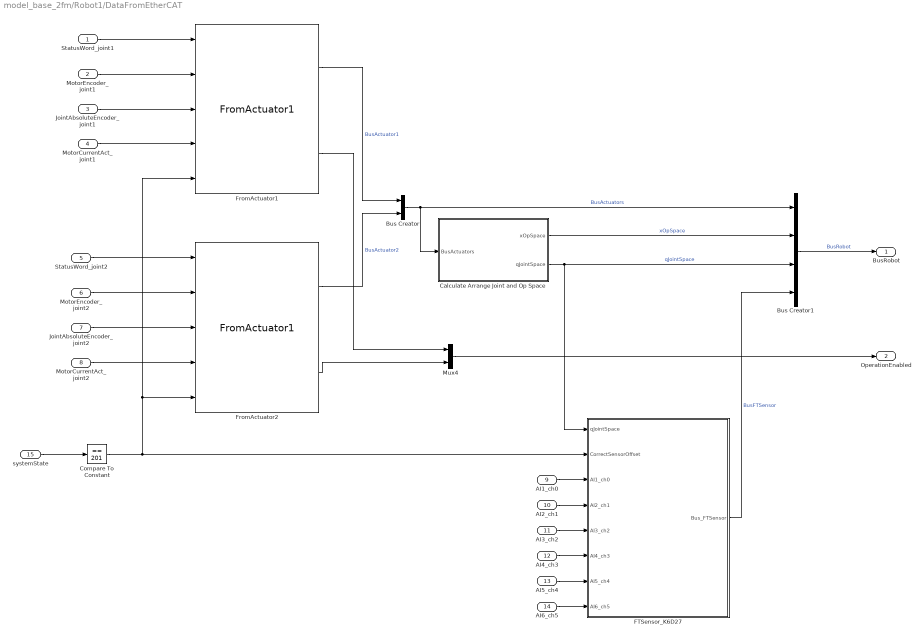
== system model_base_2fm/Robot1/DataFromEtherCAT ==
  StatusWord_joint1 : Inport
  MotorEncoder_joint1 : Inport  Port=2
  JointAbsoluteEncoder_joint1 : Inport  Port=3
  MotorCurrentAct_joint1 : Inport  Port=4
  StatusWord_joint2 : Inport  Port=5
  MotorEncoder_joint2 : Inport  Port=6
  "JointAbsoluteEncoder_joint2 " : Inport  Port=7
  MotorCurrentAct_joint2 : Inport  Port=8
  AI1_ch0 : Inport  Port=9
  AI2_ch1 : Inport  Port=10
  AI3_ch2 : Inport  Port=11
  AI4_ch3 : Inport  Port=12
  AI5_ch4 : Inport  Port=13
  AI6_ch5 : Inport  Port=14
  systemState : Inport  Port=15
  Bus Creator : BusCreator  Inputs=2
  Bus Creator1 : BusCreator  Inputs=4
  Calculate Arrange Joint and Op Space : Subsystem
  Compare To Constant : simulink/Logic and Bit Operations/Compare To Constant  relop===  const=201  OutDataTypeStr=boolean
  FTSensor_K6D27 : Subsystem  mask{FTSensorStruct=RobotStruct.FTSensor}
      mask prompts: FTSensorStruct "Struct for force torque sensor"
  FromActuator1 : LibraryFM/FromActuator1  ActuatorStruct=RobotStruct.Actuator1
  FromActuator2 : LibraryFM/FromActuator1  ActuatorStruct=RobotStruct.Actuator2
  Mux4 : Mux  Inputs=2
  BusRobot : Outport
  OperationEnabled : Outport  Port=2
  wires:
  FTSensor_K6D27/1(Bus_FTSensor) -> Bus Creator1/4  "BusFTSensor"
  FromActuator1/1 -> Bus Creator/1  "BusActuator1"
  FromActuator2/1 -> Bus Creator/2  "BusActuator2"
  FromActuator1/2 -> Mux4/1
  Mux4/1 -> OperationEnabled/1
  FromActuator2/2 -> Mux4/2
  MotorEncoder_joint1/1 -> FromActuator1/2
  StatusWord_joint1/1 -> FromActuator1/1
  JointAbsoluteEncoder_joint1/1 -> FromActuator1/3
  MotorCurrentAct_joint1/1 -> FromActuator1/4
  MotorEncoder_joint2/1 -> FromActuator2/2
  StatusWord_joint2/1 -> FromActuator2/1
  "JointAbsoluteEncoder_joint2 "/1 -> FromActuator2/3
  MotorCurrentAct_joint2/1 -> FromActuator2/4
  Bus Creator/1 -> Calculate Arrange Joint and Op Space/1(BusActuators), Bus Creator1/1  "BusActuators"
  Bus Creator1/1 -> BusRobot/1  "BusRobot"
  Calculate Arrange Joint and Op Space/2(qJointSpace) -> Bus Creator1/3, FTSensor_K6D27/1(qJointSpace)  "qJointSpace"
  systemState/1 -> Compare To Constant/1
  AI1_ch0/1 -> FTSensor_K6D27/3(AI1_ch0)
  AI2_ch1/1 -> FTSensor_K6D27/4(AI2_ch1)
  AI3_ch2/1 -> FTSensor_K6D27/5(AI3_ch2)
  AI4_ch3/1 -> FTSensor_K6D27/6(AI4_ch3)
  AI5_ch4/1 -> FTSensor_K6D27/7(AI5_ch4)
  AI6_ch5/1 -> FTSensor_K6D27/8(AI6_ch5)
  Compare To Constant/1 -> FromActuator1/5, FromActuator2/5, FTSensor_K6D27/2(CorrectSensorOffset)
  Calculate Arrange Joint and Op Space/1(xOpSpace) -> Bus Creator1/2  "xOpSpace"

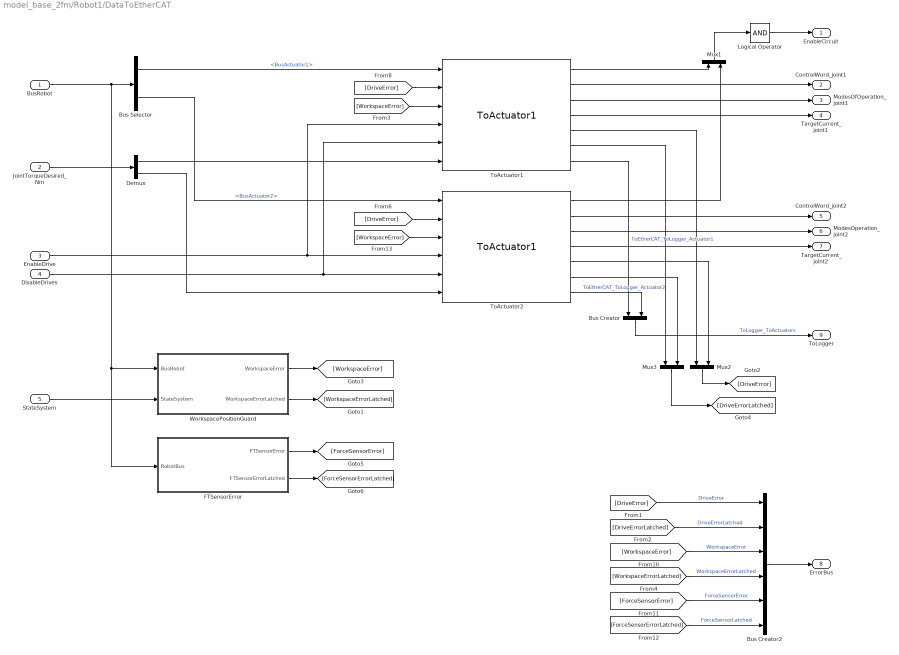
== system model_base_2fm/Robot1/DataToEtherCAT ==
  BusRobot : Inport
  JointTorqueDesired_Nm : Inport  Port=2
  EnableDrive : Inport  Port=3
  DisableDrives : Inport  Port=4
  StateSystem : Inport  Port=5
  Bus Creator : BusCreator  Inputs=2
  Bus Creator2 : BusCreator  Inputs=6
  Bus Selector : BusSelector  OutputSignals=BusActuators.BusActuator1,BusActuators.BusActuator2
  Demux : Demux  Outputs=2
  FTSensorError : Subsystem
  Logical Operator : Logic  Inputs=1  AllPortsSameDT=off  OutDataTypeStr=boolean
  Mux1 : Mux  Inputs=2
  Mux2 : Mux  Inputs=2
  Mux3 : Mux  Inputs=2
  ToActuator1 : LibraryFM/ToActuator1  ActuatorStruct=RobotStruct.Actuator1
  ToActuator2 : LibraryFM/ToActuator1  ActuatorStruct=RobotStruct.Actuator2
  WorkspacePositionGuard : Subsystem
  EnableCircuit : Outport  OutDataTypeStr=boolean
  ControlWord_joint1 : Outport  Port=2  OutDataTypeStr=uint16
  ModesOfOperation_joint1 : Outport  Port=3  OutDataTypeStr=int8
  TargetCurrent_joint1 : Outport  Port=4  OutDataTypeStr=int16
  ControlWord_joint2 : Outport  Port=5  OutDataTypeStr=uint16
  ModesOperation_joint2 : Outport  Port=6  OutDataTypeStr=int8
  TargetCurrent_joint2 : Outport  Port=7  OutDataTypeStr=int16
  ErrorBus : Outport  Port=8
  ToLogger : Outport  Port=9
  wires:
  Bus Creator/1 -> ToLogger/1  "ToLogger_ToActuators"
  ToActuator2/7 -> Bus Creator/2  "ToEtherCAT_ToLogger_Actuator2"
  ToActuator1/7 -> Bus Creator/1  "ToEtherCAT_ToLogger_Actuator1"
  ToActuator1/5 -> Mux2/1
  ToActuator2/5 -> Mux2/2
  Mux2/1 -> [DriveError]
  ToActuator1/6 -> Mux3/1
  ToActuator2/6 -> Mux3/2
  [DriveError] -> ToActuator1/2
  Mux1/1 -> Logical Operator/1
  ToActuator1/1 -> Mux1/1
  ToActuator2/1 -> Mux1/2
  ToActuator1/2 -> ControlWord_joint1/1
  ToActuator1/3 -> ModesOfOperation_joint1/1
  ToActuator2/2 -> ControlWord_joint2/1
  ToActuator1/4 -> TargetCurrent_joint1/1
  ToActuator2/4 -> TargetCurrent_joint2/1
  ToActuator2/3 -> ModesOperation_joint2/1
  Logical Operator/1 -> EnableCircuit/1
  Demux/2 -> ToActuator2/6
  JointTorqueDesired_Nm/1 -> Demux/1
  Demux/1 -> ToActuator1/6
  BusRobot/1 -> WorkspacePositionGuard/1(BusRobot), FTSensorError/1(RobotBus), Bus Selector/1
  Bus Selector/2 -> ToActuator2/1  "<BusActuator2>"
  Bus Selector/1 -> ToActuator1/1  "<BusActuator1>"
  [WorkspaceError] -> ToActuator1/3
  DisableDrives/1 -> ToActuator1/5, ToActuator2/5
  EnableDrive/1 -> ToActuator1/4, ToActuator2/4
  [DriveError] -> ToActuator2/2
  [WorkspaceError] -> ToActuator2/3
  Mux3/1 -> [DriveErrorLatched]
  Bus Creator2/1 -> ErrorBus/1
  [DriveError] -> Bus Creator2/1  "DriveError"
  [DriveErrorLatched] -> Bus Creator2/2  "DriveErrorLatched"
  [WorkspaceError] -> Bus Creator2/3  "WorkspaceError"
  [WorkspaceErrorLatched] -> Bus Creator2/4  "WorkspaceErrorLatched"
  StateSystem/1 -> WorkspacePositionGuard/2(StateSystem)
  [ForceSensorError] -> Bus Creator2/5  "ForceSensorError"
  [ForceSensorErrorLatched] -> Bus Creator2/6  "ForceSensorLatched"
  FTSensorError/1(FTSensorError) -> [ForceSensorError]
  FTSensorError/2(FTSensorErrorLatched) -> [ForceSensorErrorLatched]
  WorkspacePositionGuard/1(WorkspaceError) -> [WorkspaceError]
  WorkspacePositionGuard/2(WorkspaceErrorLatched) -> [WorkspaceErrorLatched]

== system model_base_2fm/Robot1/StateMachineLocal ==
  note: Very crude error handling
      | Ideally, the state machine gets all
      | the error codes (2,4,8, etc) such that
      | it can discern between states
  RobotBus : Inport
  reqSystemState : Inport  Port=2
  ErrorBus : Inport  Port=3
  Bus Selector : BusSelector  OutputSignals=qJointSpace.qdot,xOpSpace.x
  Bus Selector1 : BusSelector  OutputSignals=DriveError,WorkspaceError,ForceSensorError  OutputAsBus=on
  CheckVelThreshold : MATLAB Function  TreatAsAtomicUnit=on
  Compare To Constant : simulink/Logic and Bit Operations/Compare To Constant  relop=>  const=0  OutDataTypeStr=boolean
  Constant : Constant  Value=RobotStruct.HomeLocationSize
  Constant1 : Constant  Value=RobotStruct.HomeLocationOpSpace
  Constant2 : Constant  Value=0.05
  Detect Change1 : simulink/Logic and Bit Operations/Detect Change  Commented=on  vinit=0  InputProcessing=Inherited  OutDataTypeStr=boolean
  Encode system state change : MATLAB Function  Commented=on  TreatAsAtomicUnit=on
  Logical Operator : Logic  Operator=OR  Inputs=1  AllPortsSameDT=off  OutDataTypeStr=boolean
  State machine : Stateflow chart  TreatAsAtomicUnit=on
  Terminator : Terminator  Commented=on
  checkEndpointPosition : MATLAB Function  TreatAsAtomicUnit=on
  system state : Display
  currentState : Outport
  wires:
  Bus Selector1/1 -> Compare To Constant/1
  ErrorBus/1 -> Bus Selector1/1
  State machine/1(currentState) -> currentState/1, system state/1
  Logical Operator/1 -> State machine/2(fault)
  Compare To Constant/1 -> Logical Operator/1
  reqSystemState/1 -> State machine/1(requestedState)
  Detect Change1/1 -> Encode system state change/1(stateChanged)
  Encode system state change/1(systemStateChanged) -> Terminator/1
  RobotBus/1 -> Bus Selector/1
  Bus Selector/1 -> CheckVelThreshold/1(qdot)  "<qdot>"
  Bus Selector/2 -> checkEndpointPosition/1(x)  "<x>"
  CheckVelThreshold/1(velBelowThreshold) -> State machine/3(velBelowThreshold)
  Constant2/1 -> CheckVelThreshold/2(threshold)
  Constant1/1 -> checkEndpointPosition/2(homeLocation)
  Constant/1 -> checkEndpointPosition/3(threshold)
  checkEndpointPosition/1(isAtEndpoint) -> State machine/4(isAtHome)

== system model_base_2fm/Robot2/AppendToLoggerBus ==
  BusRobot : Inport
  ToEtherCAT_ToLogger : Inport  Port=2
  Controller_ToLogger : Inport  Port=3
  SystemState : Inport  Port=4
  Bus Creator : BusCreator  Inputs=8
  Bus Selector : BusSelector  OutputSignals=xOpSpace,qJointSpace,BusFTSensor,BusActuators
  Bus Selector1 : BusSelector  OutputSignals=ToEtherCAT_ToLogger_Actuator1,ToEtherCAT_ToLogger_Actuator2
  ToLogger : Outport
  wires:
  Bus Creator/1 -> ToLogger/1  "LoggerBus"
  Bus Selector/4 -> Bus Creator/4  "<BusActuators>"
  Bus Selector/1 -> Bus Creator/1  "<xOpSpace>"
  Bus Selector/3 -> Bus Creator/3  "<BusFTSensor>"
  Bus Selector/2 -> Bus Creator/2  "<qJointSpace>"
  BusRobot/1 -> Bus Selector/1
  ToEtherCAT_ToLogger/1 -> Bus Selector1/1
  Bus Selector1/1 -> Bus Creator/5  "<ToEtherCAT_ToLogger_Actuator1>"
  Bus Selector1/2 -> Bus Creator/6  "<ToEtherCAT_ToLogger_Actuator2>"
  Controller_ToLogger/1 -> Bus Creator/7
  SystemState/1 -> Bus Creator/8  "SystemState"

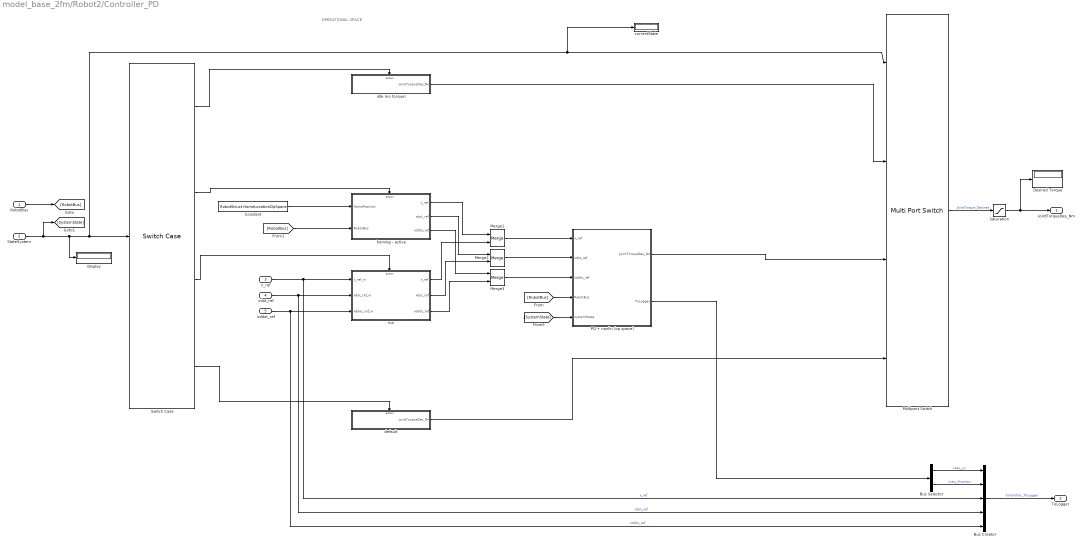
== system model_base_2fm/Robot2/Controller_PD ==
  note: OPERATIONAL SPACE
  RobotBus : Inport
  StateSystem : Inport  Port=2
  x_ref : Inport  Port=3
  xdot_ref : Inport  Port=4
  xddot_ref : Inport  Port=5
  Bus Creator : BusCreator  Inputs=5
  Bus Selector : BusSelector  OutputSignals=tau_y,tau_nlcomp
  Constant : Constant  Value=RobotStruct.HomeLocationOpSpace
  Desired Torque : Display
  Display : Display
  Merge1 : Merge  InitialOutput=[0;0]
  Merge2 : Merge  InitialOutput=[0;0]
  Merge3 : Merge  InitialOutput=[0;0]
  Multiport Switch : MultiPortSwitch  DataPortOrder=Specify indices  Inputs=4  DataPortIndices={[0,1,2,201,299,301],[302,399,4]}  DataPortForDefault=Additional data port
  PD + nonlin (op space) : Subsystem
  Saturation : Saturate  UpperLimit=4  LowerLimit=-4
  Switch Case : SwitchCase  CaseConditions={[0,1,2,201,299,301],[302, 399],[4]}
  currentState : Display
  default : Subsystem  TreatAsAtomicUnit=on
  homing - active : Subsystem
  idle (no torque) : Subsystem  TreatAsAtomicUnit=on
  run : Subsystem
  JointTorqueDes_Nm : Outport
  ToLogger : Outport  Port=2
  wires:
  [SystemState] -> PD + nonlin (op space)/5(systemState)
  xddot_ref/1 -> Bus Creator/5, run/3(xddot_ref_in)  "xddot_ref"
  xdot_ref/1 -> Bus Creator/4, run/2(xdot_ref_in)  "xdot_ref"
  x_ref/1 -> Bus Creator/3, run/1(x_ref_in)  "x_ref"
  [RobotBus] -> homing - active/2(RobotBus)
  [RobotBus] -> PD + nonlin (op space)/4(RobotBus)
  RobotBus/1 -> [RobotBus]
  PD + nonlin (op space)/1(JointTorqueDes_Nm) -> Multiport Switch/3
  Merge3/1 -> PD + nonlin (op space)/3(xddot_ref)
  Merge2/1 -> PD + nonlin (op space)/2(xdot_ref)
  Merge1/1 -> PD + nonlin (op space)/1(x_ref)
  idle (no torque)/1(JointTorqueDes_Nm) -> Multiport Switch/2
  Switch Case/2 -> homing - active/Action
  Switch Case/1 -> idle (no torque)/Action
  default/1(JointTorqueDes_Nm) -> Multiport Switch/4
  Switch Case/4 -> default/Action
  Saturation/1 -> Desired Torque/1, JointTorqueDes_Nm/1
  Switch Case/3 -> run/Action
  homing - active/1(x_ref) -> Merge1/1
  run/1(x_ref) -> Merge1/2
  StateSystem/1 -> Display/1, Multiport Switch/1, currentState/1, Switch Case/1, [SystemState]
  run/2(xdot_ref) -> Merge2/2
  run/3(xddot_ref) -> Merge3/2
  homing - active/2(xdot_ref) -> Merge2/1
  homing - active/3(xddot_ref) -> Merge3/1
  Multiport Switch/1 -> Saturation/1  "JointTorque_Desired"
  PD + nonlin (op space)/2(ToLogger) -> Bus Selector/1
  Constant/1 -> homing - active/1(HomePosition)
  Bus Creator/1 -> ToLogger/1  "Controller_ToLogger"
  Bus Selector/1 -> Bus Creator/1  "<tau_y>"
  Bus Selector/2 -> Bus Creator/2  "<tau_nlcomp>"

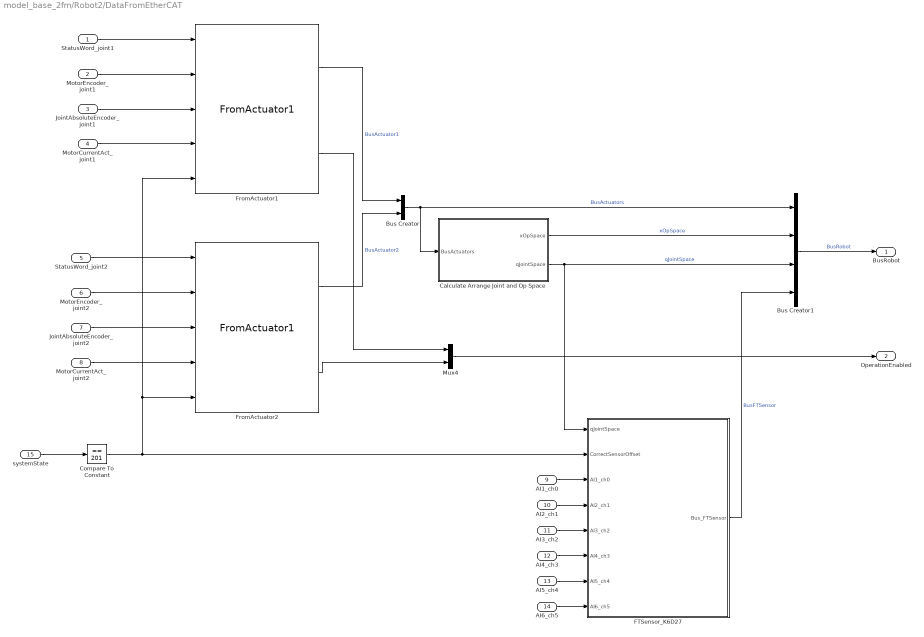
== system model_base_2fm/Robot2/DataFromEtherCAT ==
  StatusWord_joint1 : Inport
  MotorEncoder_joint1 : Inport  Port=2
  JointAbsoluteEncoder_joint1 : Inport  Port=3
  MotorCurrentAct_joint1 : Inport  Port=4
  StatusWord_joint2 : Inport  Port=5
  MotorEncoder_joint2 : Inport  Port=6
  "JointAbsoluteEncoder_joint2 " : Inport  Port=7
  MotorCurrentAct_joint2 : Inport  Port=8
  AI1_ch0 : Inport  Port=9
  AI2_ch1 : Inport  Port=10
  AI3_ch2 : Inport  Port=11
  AI4_ch3 : Inport  Port=12
  AI5_ch4 : Inport  Port=13
  AI6_ch5 : Inport  Port=14
  systemState : Inport  Port=15
  Bus Creator : BusCreator  Inputs=2
  Bus Creator1 : BusCreator  Inputs=4
  Calculate Arrange Joint and Op Space : Subsystem
  Compare To Constant : simulink/Logic and Bit Operations/Compare To Constant  relop===  const=201  OutDataTypeStr=boolean
  FTSensor_K6D27 : Subsystem  mask{FTSensorStruct=RobotStruct.FTSensor}
      mask prompts: FTSensorStruct "Struct for force torque sensor"
  FromActuator1 : LibraryFM/FromActuator1  ActuatorStruct=RobotStruct.Actuator1
  FromActuator2 : LibraryFM/FromActuator1  ActuatorStruct=RobotStruct.Actuator2
  Mux4 : Mux  Inputs=2
  BusRobot : Outport
  OperationEnabled : Outport  Port=2
  wires:
  FTSensor_K6D27/1(Bus_FTSensor) -> Bus Creator1/4  "BusFTSensor"
  FromActuator1/1 -> Bus Creator/1  "BusActuator1"
  FromActuator2/1 -> Bus Creator/2  "BusActuator2"
  FromActuator1/2 -> Mux4/1
  Mux4/1 -> OperationEnabled/1
  FromActuator2/2 -> Mux4/2
  MotorEncoder_joint1/1 -> FromActuator1/2
  StatusWord_joint1/1 -> FromActuator1/1
  JointAbsoluteEncoder_joint1/1 -> FromActuator1/3
  MotorCurrentAct_joint1/1 -> FromActuator1/4
  MotorEncoder_joint2/1 -> FromActuator2/2
  StatusWord_joint2/1 -> FromActuator2/1
  "JointAbsoluteEncoder_joint2 "/1 -> FromActuator2/3
  MotorCurrentAct_joint2/1 -> FromActuator2/4
  Bus Creator/1 -> Calculate Arrange Joint and Op Space/1(BusActuators), Bus Creator1/1  "BusActuators"
  Bus Creator1/1 -> BusRobot/1  "BusRobot"
  Calculate Arrange Joint and Op Space/2(qJointSpace) -> Bus Creator1/3, FTSensor_K6D27/1(qJointSpace)  "qJointSpace"
  systemState/1 -> Compare To Constant/1
  AI1_ch0/1 -> FTSensor_K6D27/3(AI1_ch0)
  AI2_ch1/1 -> FTSensor_K6D27/4(AI2_ch1)
  AI3_ch2/1 -> FTSensor_K6D27/5(AI3_ch2)
  AI4_ch3/1 -> FTSensor_K6D27/6(AI4_ch3)
  AI5_ch4/1 -> FTSensor_K6D27/7(AI5_ch4)
  AI6_ch5/1 -> FTSensor_K6D27/8(AI6_ch5)
  Compare To Constant/1 -> FromActuator1/5, FromActuator2/5, FTSensor_K6D27/2(CorrectSensorOffset)
  Calculate Arrange Joint and Op Space/1(xOpSpace) -> Bus Creator1/2  "xOpSpace"

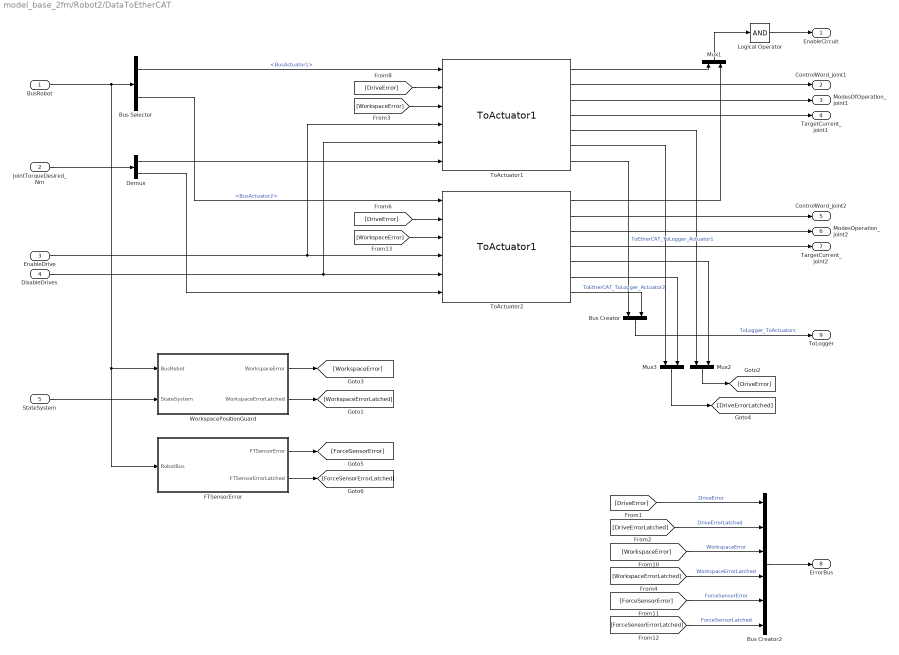
== system model_base_2fm/Robot2/DataToEtherCAT ==
  BusRobot : Inport
  JointTorqueDesired_Nm : Inport  Port=2
  EnableDrive : Inport  Port=3
  DisableDrives : Inport  Port=4
  StateSystem : Inport  Port=5
  Bus Creator : BusCreator  Inputs=2
  Bus Creator2 : BusCreator  Inputs=6
  Bus Selector : BusSelector  OutputSignals=BusActuators.BusActuator1,BusActuators.BusActuator2
  Demux : Demux  Outputs=2
  FTSensorError : Subsystem
  Logical Operator : Logic  Inputs=1  AllPortsSameDT=off  OutDataTypeStr=boolean
  Mux1 : Mux  Inputs=2
  Mux2 : Mux  Inputs=2
  Mux3 : Mux  Inputs=2
  ToActuator1 : LibraryFM/ToActuator1  ActuatorStruct=RobotStruct.Actuator1
  ToActuator2 : LibraryFM/ToActuator1  ActuatorStruct=RobotStruct.Actuator2
  WorkspacePositionGuard : Subsystem
  EnableCircuit : Outport  OutDataTypeStr=boolean
  ControlWord_joint1 : Outport  Port=2  OutDataTypeStr=uint16
  ModesOfOperation_joint1 : Outport  Port=3  OutDataTypeStr=int8
  TargetCurrent_joint1 : Outport  Port=4  OutDataTypeStr=int16
  ControlWord_joint2 : Outport  Port=5  OutDataTypeStr=uint16
  ModesOperation_joint2 : Outport  Port=6  OutDataTypeStr=int8
  TargetCurrent_joint2 : Outport  Port=7  OutDataTypeStr=int16
  ErrorBus : Outport  Port=8
  ToLogger : Outport  Port=9
  wires:
  Bus Creator/1 -> ToLogger/1  "ToLogger_ToActuators"
  ToActuator2/7 -> Bus Creator/2  "ToEtherCAT_ToLogger_Actuator2"
  ToActuator1/7 -> Bus Creator/1  "ToEtherCAT_ToLogger_Actuator1"
  ToActuator1/5 -> Mux2/1
  ToActuator2/5 -> Mux2/2
  Mux2/1 -> [DriveError]
  ToActuator1/6 -> Mux3/1
  ToActuator2/6 -> Mux3/2
  [DriveError] -> ToActuator1/2
  Mux1/1 -> Logical Operator/1
  ToActuator1/1 -> Mux1/1
  ToActuator2/1 -> Mux1/2
  ToActuator1/2 -> ControlWord_joint1/1
  ToActuator1/3 -> ModesOfOperation_joint1/1
  ToActuator2/2 -> ControlWord_joint2/1
  ToActuator1/4 -> TargetCurrent_joint1/1
  ToActuator2/4 -> TargetCurrent_joint2/1
  ToActuator2/3 -> ModesOperation_joint2/1
  Logical Operator/1 -> EnableCircuit/1
  Demux/2 -> ToActuator2/6
  JointTorqueDesired_Nm/1 -> Demux/1
  Demux/1 -> ToActuator1/6
  BusRobot/1 -> WorkspacePositionGuard/1(BusRobot), FTSensorError/1(RobotBus), Bus Selector/1
  Bus Selector/2 -> ToActuator2/1  "<BusActuator2>"
  Bus Selector/1 -> ToActuator1/1  "<BusActuator1>"
  [WorkspaceError] -> ToActuator1/3
  DisableDrives/1 -> ToActuator1/5, ToActuator2/5
  EnableDrive/1 -> ToActuator1/4, ToActuator2/4
  [DriveError] -> ToActuator2/2
  [WorkspaceError] -> ToActuator2/3
  Mux3/1 -> [DriveErrorLatched]
  Bus Creator2/1 -> ErrorBus/1
  [DriveError] -> Bus Creator2/1  "DriveError"
  [DriveErrorLatched] -> Bus Creator2/2  "DriveErrorLatched"
  [WorkspaceError] -> Bus Creator2/3  "WorkspaceError"
  [WorkspaceErrorLatched] -> Bus Creator2/4  "WorkspaceErrorLatched"
  StateSystem/1 -> WorkspacePositionGuard/2(StateSystem)
  [ForceSensorError] -> Bus Creator2/5  "ForceSensorError"
  [ForceSensorErrorLatched] -> Bus Creator2/6  "ForceSensorLatched"
  FTSensorError/1(FTSensorError) -> [ForceSensorError]
  FTSensorError/2(FTSensorErrorLatched) -> [ForceSensorErrorLatched]
  WorkspacePositionGuard/1(WorkspaceError) -> [WorkspaceError]
  WorkspacePositionGuard/2(WorkspaceErrorLatched) -> [WorkspaceErrorLatched]
